simulink model "Additional"  (R2012b)
settings: Solver=ode45  StartTime=0.0  StopTime=10.0  RelTol=1e-3
settings Model: Creator=tth-sza  LastModifiedBy=tth-sza

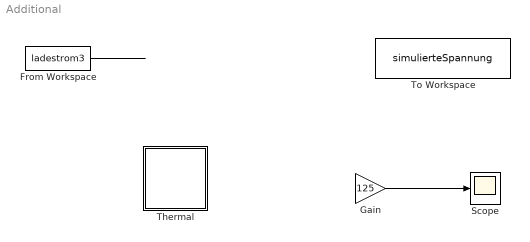
== system Additional ==
  From Workspace : FromWorkspace  VariableName=ladestrom3  SampleTime=0
  Gain : Gain  Gain=125
  Scope : Scope
      settings: TimeRange=200
  Thermal : Subsystem
  To Workspace : ToWorkspace  VariableName=simulierteSpannung  SampleTime=-1  SaveFormat=Structure With Time
  wires:
  From Workspace/1 -> ?
  ? -> Gain/1, To Workspace/1
  Gain/1 -> Scope/1

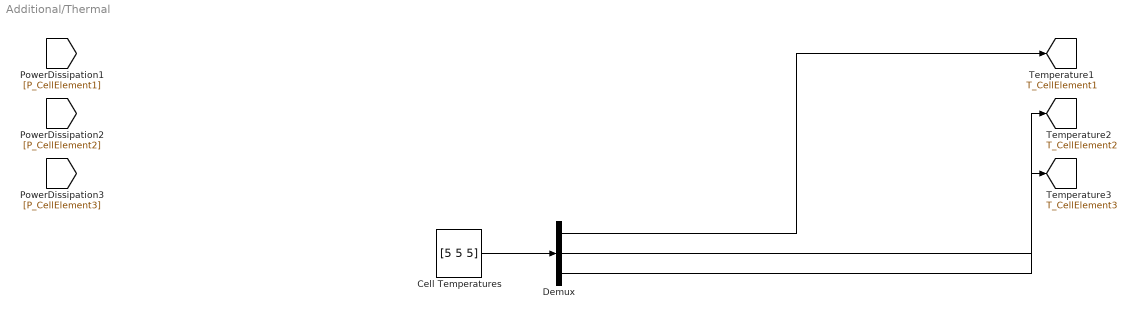
== system Additional/Thermal ==
  Cell Temperatures : Constant  Value=[5 5 5]
  Demux : Demux  Outputs=3
  tag scope: T_CellElement1=global, T_CellElement2=global, T_CellElement3=global
  wires:
  Cell Temperatures/1 -> Demux/1
  Demux/1 -> [T_CellElement1]
  Demux/2 -> [T_CellElement2]
  Demux/3 -> [T_CellElement3]
